simulink model "HinfDesign1_nodev"  (R2018b)
settings: Solver=VariableStepAuto  StartTime=0.0  StopTime=200  RelTol=1e-3
model workspace: external: MATLAB File C:\Users\Yavuz\Documents\MATLAB\constants.m (data not in the file)
values from neighbouring files (symbols this model uses):
  alpha = 0.5736    [constants.m]
  c_damp = 0.00495    [constants.m]
  in_nu = 0.0001    [constants.m]
  J_s = 31.38    [constants.m]
  time_cons = 0.5    [constants.m]
  w_mode = 2.6268    [constants.m]
settings Model: Creator=Yavuz  LastModifiedBy=Yavuz
settings DebuggingCC: AlgebraicLoopMsg=none

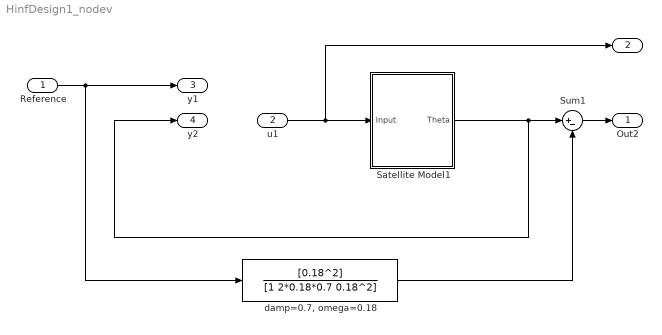
== system HinfDesign1_nodev ==
  Reference : Inport
  u1 : Inport  Port=2
  Satellite Model1 : Subsystem
  Sum1 : Sum  Inputs=|+-
  "damp=0.7, omega=0.18" : TransferFcn  Numerator=[0.18^2]  Denominator=[1 2*0.18*0.7 0.18^2]
  Out2 : Outport
  " " : Outport  Port=2
  y1 : Outport  Port=3
  y2 : Outport  Port=4
  wires:
  u1/1 -> Satellite Model1/1(Input), " "/1
  Sum1/1 -> Out2/1
  "damp=0.7, omega=0.18"/1 -> Sum1/2
  Reference/1 -> y1/1, "damp=0.7, omega=0.18"/1
  Satellite Model1/1(Theta) -> Sum1/1, y2/1

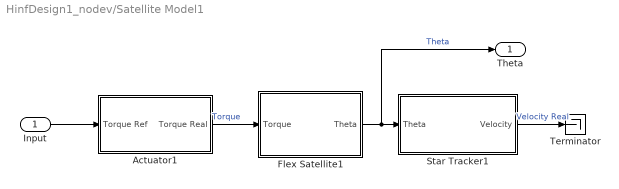
== system HinfDesign1_nodev/Satellite Model1 ==
  Input : Inport
  Actuator1 : Subsystem
  Flex Satellite1 : Subsystem
  Star Tracker1 : Subsystem
  Terminator : Terminator
  Theta : Outport
  wires:
  Actuator1/1(Torque Real) -> Flex Satellite1/1(Torque)  "Torque"
  Flex Satellite1/1(Theta) -> Theta/1, Star Tracker1/1(Theta)  "Theta"
  Input/1 -> Actuator1/1(Torque Ref)
  Star Tracker1/1(Velocity) -> Terminator/1  "Velocity Real"

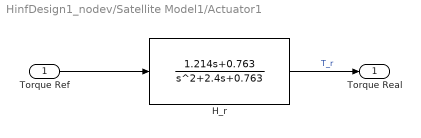
== system HinfDesign1_nodev/Satellite Model1/Actuator1 ==
  Torque Ref : Inport
  H_r : TransferFcn  Numerator=[1.214 0.763]  Denominator=[1 2.4 0.763]
  Torque Real : Outport
  wires:
  Torque Ref/1 -> H_r/1
  H_r/1 -> Torque Real/1  "T_r"

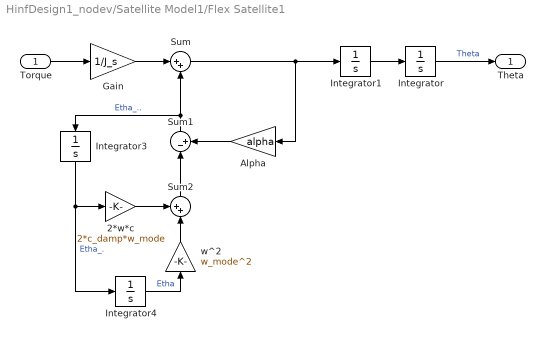
== system HinfDesign1_nodev/Satellite Model1/Flex Satellite1 ==
  Torque : Inport
  2*w*c : Gain  Gain=2*c_damp*w_mode
  Alpha : Gain  Gain=alpha
  Gain : Gain  Gain=1/J_s
  Integrator : Integrator
  Integrator1 : Integrator
  Integrator3 : Integrator
  Integrator4 : Integrator  InitialCondition=in_nu
  Sum : Sum  Inputs=|++
  Sum1 : Sum  Inputs=|-+
  Sum2 : Sum  Inputs=++|
  w^2 : Gain  Gain=w_mode^2
  Theta : Outport
  wires:
  Sum/1 -> Integrator1/1, Alpha/1
  Sum1/1 -> Integrator3/1, Sum/2  "Etha_.."
  Gain/1 -> Sum/1
  Integrator1/1 -> Integrator/1
  Integrator3/1 -> Integrator4/1, 2*w*c/1  "Etha_."
  Sum2/1 -> Sum1/1
  Torque/1 -> Gain/1
  2*w*c/1 -> Sum2/1
  Integrator/1 -> Theta/1  "Theta"
  w^2/1 -> Sum2/2
  Integrator4/1 -> w^2/1  "Etha"
  Alpha/1 -> Sum1/2

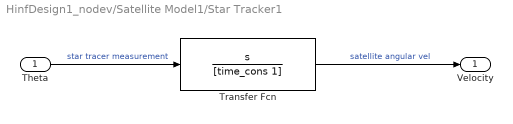
== system HinfDesign1_nodev/Satellite Model1/Star Tracker1 ==
  Theta : Inport
  Transfer Fcn : TransferFcn  Numerator=[1 0]  Denominator=[time_cons 1]
  Velocity : Outport
  wires:
  Theta/1 -> Transfer Fcn/1  "star tracer measurement"
  Transfer Fcn/1 -> Velocity/1  "satellite angular vel"
